simulink model "invkin_man"  (R2014a)
settings: Solver=ode45  StartTime=0.0  StopTime=30  FixedStep=0.01  RelTol=1e-3
PreLoadFcn:
  | fprintf('*** Loading Puma560 model to workspace\n');
  | mdl_puma560
undefined symbols (not defined in the file): DiscIntNeverNeededParam, p560, prefDir, qn, tr2rpy, transl
libraries: roblocks x6, edolib x1, dspmtrx3 x1, simulink x1
settings Model: NumberOfSteps=50  ExtModeTrigMode=oneshot  ExtModeArmWhenConnect=off  Creator=pic  LastModifiedBy=Edoardo
settings DataIOCC: LimitDataPoints=off  SignalLoggingSaveFormat=ModelDataLogs
settings OptimizationCC: BlockReduction=off  BooleanDataType=off  ExpressionDepthLimit=2147483647  InitFltsAndDblsToZero=on
settings DebuggingCC: SaveWithParameterizedLinksMsg=none  UnderspecifiedInitializationDetection=Classic  SignalResolutionControl=TryResolveAllWithWarning  SolverPrmCheckMsg=none  MultiTaskDSMMsg=warning  MultiTaskCondExecSysMsg=none  FcnCallInpInsideContextMsg=UseLocalSettings  StateNameClashWarn=warning
settings HardwareCC: TargetUnknown=on
settings RTWCC: IncludeERTFirstTime=on
settings GRTTargetCC: ModelReferenceCompliant=off  CompOptLevelCompliant=off  CombineOutputUpdateFcns=off  MatFileLogging=off  GRTInterface=on

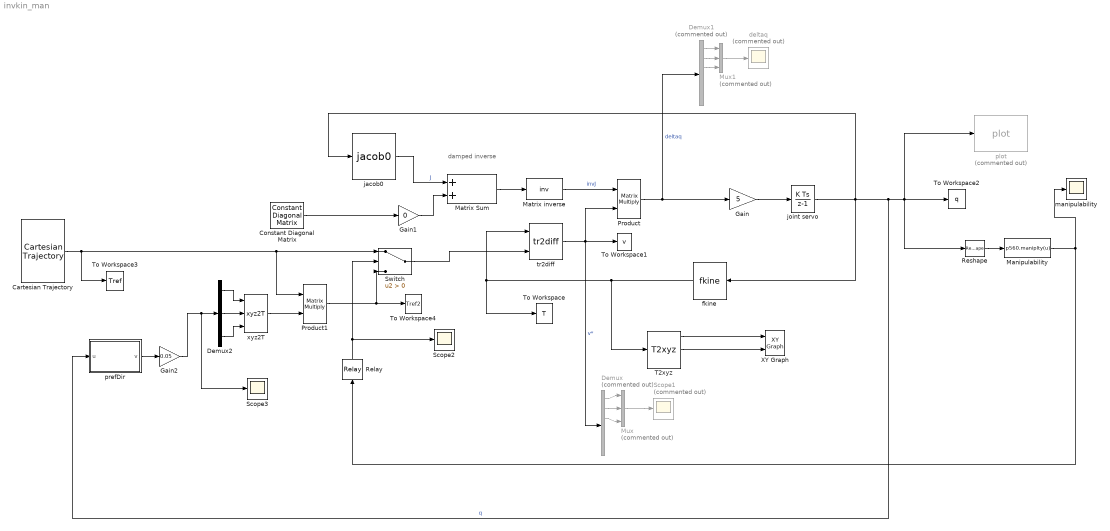
== system invkin_man ==
  note: damped inverse
  Cartesian Trajectory : edolib/Cartesian  Trajectory  ref=Internal  x0=transl(p560.fkine(qn))  rpy0=tr2rpy(p560.fkine(qn))  xf=[0.5 0.5 0]  rpyf=[0 0 0]  Tmax=30  Ts=0.2
  Constant Diagonal Matrix : dspmtrx3/Constant Diagonal Matrix  q=ones(1,6)  frame=off  dataType=Inherit from 'Constant(s) along diagonal'  isSigned=on  wordLen=16  udDataType=sfix(16)  fracBitsMode=Best precision  numFracBits=15
  Demux : Demux  Commented=on  Outputs=6
  Demux1 : Demux  Commented=on  Outputs=6
  Demux2 : Demux  Outputs=3
  Gain : Gain  Gain=5  SaturateOnIntegerOverflow=on  OutDataTypeStr=Inherit: Same as input  ParamDataTypeStr=Inherit: Same as input
  Gain1 : Gain  Gain=0
  Gain2 : Gain  Gain=0.05
  Manipulability : MATLABFcn  MATLABFcn=p560.maniplty(u)  OutputDimensions=1  Output1D=off
  Matrix Sum : Sum
  Matrix inverse : MATLABFcn  MATLABFcn=inv  Output1D=off
  Mux : Mux  Commented=on  Inputs=3
  Mux1 : Mux  Commented=on  Inputs=3
  Product : Product  Multiplication=Matrix(*)  SaturateOnIntegerOverflow=on  RndMeth=Zero  InputSameDT=on  OutDataTypeStr=Inherit: Same as first input
  Product1 : Product  Multiplication=Matrix(*)  SaturateOnIntegerOverflow=on  RndMeth=Zero  InputSameDT=on  OutDataTypeStr=Inherit: Same as first input
  Relay : Relay  OnSwitchValue=1  OffSwitchValue=0.05  OffOutputValue=-1
  Reshape : Reshape  OutputDimensionality=Row vector (2-D)
  Scope1 : Scope  Commented=on
      settings: YMin=-0.2  YMax=0.1
  Scope2 : Scope
      settings: YMin=1  YMax=1  SaveName=ScopeData3
  Scope3 : Scope
      settings: YMin=0.95  YMax=1.05  SaveName=ScopeData4
  Switch : Switch  Criteria=u2 > Threshold
  T2xyz : roblocks/Transform Conversion/T2xyz
  To Workspace : ToWorkspace  VariableName=T  SampleTime=-1
  To Workspace1 : ToWorkspace  VariableName=v  SampleTime=-1
  To Workspace2 : ToWorkspace  VariableName=q  SampleTime=-1
  To Workspace3 : ToWorkspace  VariableName=Tref  SampleTime=-1
  To Workspace4 : ToWorkspace  VariableName=Tref2  SampleTime=-1
  XY Graph : simulink/Sinks/XY Graph  xmin=-1  xmax=1  ymin=-1  ymax=1  st=-1
  deltaq : Scope  Commented=on
      settings: YMin=-0.2  YMax=0.1  SaveName=ScopeData2
  fkine : roblocks/Kinematics/fkine  robot=p560
  "jacob0 " : roblocks/Kinematics/jacob0   robot=p560
  joint servo : DiscreteIntegrator  InitialCondition=qn'  SampleTime=0.05  ICPrevOutput=DiscIntNeverNeededParam  ICPrevScaledInput=DiscIntNeverNeededParam
  manipulability : Scope
      settings: YMin=0.005  YMax=0.115
  plot : roblocks/Robot Graphics/plot  Commented=on  robot=p560  fps=25  holdplot=on
  prefDir : Subsystem  mask{r=p560}
      mask prompts: r "Robot object"
  tr2diff : roblocks/Kinematics/tr2diff  robot=p560
  xyz2T : roblocks/Transform Conversion/xyz2T
  wires:
  joint servo/1 -> "jacob0 "/1, fkine/1, prefDir/1(u), Reshape/1, plot/1, To Workspace2/1  "q"
  T2xyz/1 -> XY Graph/1
  T2xyz/2 -> XY Graph/2
  tr2diff/1 -> Demux/1, Product/2, To Workspace1/1  "v*"
  Product/1 -> Demux1/1, Gain/1  "deltaq"
  Matrix inverse/1 -> Product/1  "invJ"
  fkine/1 -> T2xyz/1, To Workspace/1, tr2diff/1
  Cartesian Trajectory/1 -> Switch/1, Product1/1, To Workspace3/1
  Manipulability/1 -> Relay/1, manipulability/1
  Reshape/1 -> Manipulability/1
  Constant Diagonal Matrix/1 -> Gain1/1
  Gain1/1 -> Matrix Sum/2
  "jacob0 "/1 -> Matrix Sum/1  "J"
  Matrix Sum/1 -> Matrix inverse/1
  Gain/1 -> joint servo/1
  Mux/1 -> Scope1/1
  Demux/1 -> Mux/1
  Demux/2 -> Mux/2
  Demux/3 -> Mux/3
  Mux1/1 -> deltaq/1
  Demux1/1 -> Mux1/1
  Demux1/2 -> Mux1/2
  Demux1/3 -> Mux1/3
  Switch/1 -> tr2diff/2
  Product1/1 -> To Workspace4/1, Switch/3
  xyz2T/1 -> Product1/2
  Relay/1 -> Scope2/1, Switch/2
  prefDir/1(v) -> Gain2/1
  Demux2/2 -> xyz2T/2
  Demux2/3 -> xyz2T/3
  Demux2/1 -> xyz2T/1
  Gain2/1 -> Scope3/1, Demux2/1

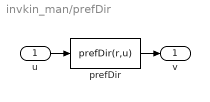
== system invkin_man/prefDir ==
  u : Inport
  "prefDir " : MATLABFcn  MATLABFcn=prefDir(r,u)  OutputDimensions=3  Output1D=off
  v : Outport
  wires:
  u/1 -> "prefDir "/1
  "prefDir "/1 -> v/1
